simulink model "CryoDetXray"  (R2016b)
settings: Solver=ode45  StartTime=0.0  StopTime=10e-5  MaxStep=Tclk/4  RelTol=1e-3
values from neighbouring files (symbols this model uses):
  Fclk = Fadc    (= 307200000)    [setupCryoFPGAxray.m]
  Tclk = 1/Fclk    (= 3.25520833333e-09)    [setupCryoFPGAxray.m]
undefined symbols (not defined in the file or in its folder): AXI4, Lite, lpf, Naxi, xlipgetpartsetting
libraries: xbsIndex_r4 x1091, CryoDetLib x68, simulink x4, hdlsllib x1
(part 2 of 8)

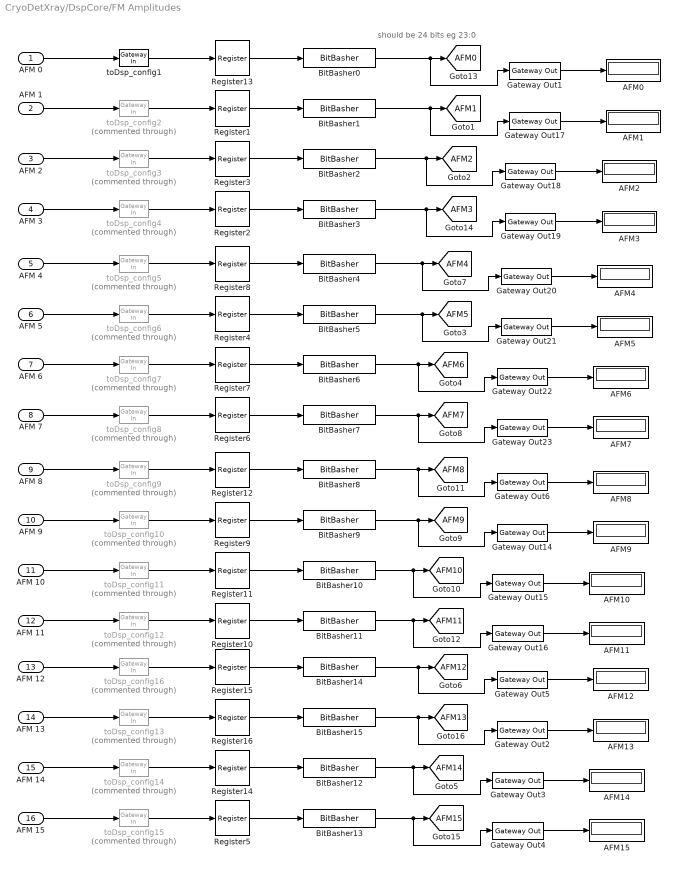
== system CryoDetXray/DspCore/FM Amplitudes ==
  note: should be 24 bits eg 23:0
  AFM 0 : Inport
  AFM 1 : Inport  Port=2
  AFM 2 : Inport  Port=3
  AFM 3 : Inport  Port=4
  AFM 4 : Inport  Port=5
  AFM 5 : Inport  Port=6
  AFM 6 : Inport  Port=7
  AFM 7 : Inport  Port=8
  AFM 8 : Inport  Port=9
  AFM 9 : Inport  Port=10
  AFM 10 : Inport  Port=11
  AFM 11 : Inport  Port=12
  AFM 12 : Inport  Port=13
  AFM 13 : Inport  Port=14
  AFM 14 : Inport  Port=15
  AFM 15 : Inport  Port=16
  AFM{0..5,7,9..15} (14 alike) : Display
  "AFM6 " : Display
  "AFM8 " : Display
  BitBasher{0..15} (16 alike) : xbsIndex_r4/BitBasher  bitexpr=a={b[23:0]}  display_expr=on  sr_1=a  arith_type1=Unsigned  bin_pt1=24  sr_2=2  arith_type2=Unsigned  bin_pt2=0  sr_3=3  arith_type3=Unsigned  bin_pt3=0  sr_4=4  arith_type4=Unsigned  bin_pt4=0  dbl_ovrd=off  block_type=bitbasher
  Gateway Out{1..6,14..23} (16 alike) : xbsIndex_r4/Gateway Out  inherit_from_input=on  hdl_port=off  rows=1  columns=1  UseAsDAC=off  DACChannel='1'  interface=None  automatic_assignment=on  address_offset=hex2dec('00')  intf_name=''  intf_description=''  timing_constraint=None  locs_specified=off  LOCs={}  io_standard={}  block_type=gatewayout
  Register{1..16} (16 alike) : xbsIndex_r4/Register  init=0  rst=off  en=off  dbl_ovrd=off  block_type=register
  toDsp_config1 : xbsIndex_r4/Gateway In  gui_display_data_type=Fixed-point  arith_type=Unsigned  n_bits=32  bin_pt=0  preci_type=Single  exp_width=8  frac_width=24  rows=1  columns=1  quantization=Truncate  overflow=Wrap  period=Tclk*Naxi  UseAsADC=off  ADCChannel='1'  interface=AXI4-Lite  automatic_assignment=off  address_offset=hex2dec('A00')  intf_name=''  intf_description=''  default_value=0  timing_constraint=None  locs_specified=off  LOCs={}  io_standard={}  inherit_from_input=off  hdl_port=on  dbl_ovrd=off  block_type=gatewayin
  toDsp_config10 : xbsIndex_r4/Gateway In  Commented=through  gui_display_data_type=Fixed-point  arith_type=Unsigned  n_bits=32  bin_pt=0  preci_type=Single  exp_width=8  frac_width=24  rows=1  columns=1  quantization=Truncate  overflow=Wrap  period=Tclk*Naxi  UseAsADC=off  ADCChannel='1'  interface=AXI4-Lite  automatic_assignment=off  address_offset=hex2dec('A24')  intf_name=''  intf_description=''  default_value=0  timing_constraint=None  locs_specified=off  LOCs={}  io_standard={}  inherit_from_input=off  hdl_port=on  dbl_ovrd=off  block_type=gatewayin
  toDsp_config11 : xbsIndex_r4/Gateway In  Commented=through  gui_display_data_type=Fixed-point  arith_type=Unsigned  n_bits=32  bin_pt=0  preci_type=Single  exp_width=8  frac_width=24  rows=1  columns=1  quantization=Truncate  overflow=Wrap  period=Tclk*Naxi  UseAsADC=off  ADCChannel='1'  interface=AXI4-Lite  automatic_assignment=off  address_offset=hex2dec('A28')  intf_name=''  intf_description=''  default_value=0  timing_constraint=None  locs_specified=off  LOCs={}  io_standard={}  inherit_from_input=off  hdl_port=on  dbl_ovrd=off  block_type=gatewayin
  toDsp_config12 : xbsIndex_r4/Gateway In  Commented=through  gui_display_data_type=Fixed-point  arith_type=Unsigned  n_bits=32  bin_pt=0  preci_type=Single  exp_width=8  frac_width=24  rows=1  columns=1  quantization=Truncate  overflow=Wrap  period=Tclk*Naxi  UseAsADC=off  ADCChannel='1'  interface=AXI4-Lite  automatic_assignment=off  address_offset=hex2dec('A2c')  intf_name=''  intf_description=''  default_value=0  timing_constraint=None  locs_specified=off  LOCs={}  io_standard={}  inherit_from_input=off  hdl_port=on  dbl_ovrd=off  block_type=gatewayin
  toDsp_config13 : xbsIndex_r4/Gateway In  Commented=through  gui_display_data_type=Fixed-point  arith_type=Unsigned  n_bits=32  bin_pt=0  preci_type=Single  exp_width=8  frac_width=24  rows=1  columns=1  quantization=Truncate  overflow=Wrap  period=Tclk*Naxi  UseAsADC=off  ADCChannel='1'  interface=AXI4-Lite  automatic_assignment=off  address_offset=hex2dec('A34')  intf_name=''  intf_description=''  default_value=0  timing_constraint=None  locs_specified=off  LOCs={}  io_standard={}  inherit_from_input=off  hdl_port=on  dbl_ovrd=off  block_type=gatewayin
  toDsp_config14 : xbsIndex_r4/Gateway In  Commented=through  gui_display_data_type=Fixed-point  arith_type=Unsigned  n_bits=32  bin_pt=0  preci_type=Single  exp_width=8  frac_width=24  rows=1  columns=1  quantization=Truncate  overflow=Wrap  period=Tclk*Naxi  UseAsADC=off  ADCChannel='1'  interface=AXI4-Lite  automatic_assignment=off  address_offset=hex2dec('A38')  intf_name=''  intf_description=''  default_value=0  timing_constraint=None  locs_specified=off  LOCs={}  io_standard={}  inherit_from_input=off  hdl_port=on  dbl_ovrd=off  block_type=gatewayin
  toDsp_config15 : xbsIndex_r4/Gateway In  Commented=through  gui_display_data_type=Fixed-point  arith_type=Unsigned  n_bits=32  bin_pt=0  preci_type=Single  exp_width=8  frac_width=24  rows=1  columns=1  quantization=Truncate  overflow=Wrap  period=Tclk*Naxi  UseAsADC=off  ADCChannel='1'  interface=AXI4-Lite  automatic_assignment=off  address_offset=hex2dec('A3c')  intf_name=''  intf_description=''  default_value=0  timing_constraint=None  locs_specified=off  LOCs={}  io_standard={}  inherit_from_input=off  hdl_port=on  dbl_ovrd=off  block_type=gatewayin
  toDsp_config16 : xbsIndex_r4/Gateway In  Commented=through  gui_display_data_type=Fixed-point  arith_type=Unsigned  n_bits=32  bin_pt=0  preci_type=Single  exp_width=8  frac_width=24  rows=1  columns=1  quantization=Truncate  overflow=Wrap  period=Tclk*Naxi  UseAsADC=off  ADCChannel='1'  interface=AXI4-Lite  automatic_assignment=off  address_offset=hex2dec('A30')  intf_name=''  intf_description=''  default_value=0  timing_constraint=None  locs_specified=off  LOCs={}  io_standard={}  inherit_from_input=off  hdl_port=on  dbl_ovrd=off  block_type=gatewayin
  toDsp_config2 : xbsIndex_r4/Gateway In  Commented=through  gui_display_data_type=Fixed-point  arith_type=Unsigned  n_bits=32  bin_pt=0  preci_type=Single  exp_width=8  frac_width=24  rows=1  columns=1  quantization=Truncate  overflow=Wrap  period=Tclk*Naxi  UseAsADC=off  ADCChannel='1'  interface=AXI4-Lite  automatic_assignment=off  address_offset=hex2dec('A04')  intf_name=''  intf_description=''  default_value=0  timing_constraint=None  locs_specified=off  LOCs={}  io_standard={}  inherit_from_input=off  hdl_port=on  dbl_ovrd=off  block_type=gatewayin
  toDsp_config3 : xbsIndex_r4/Gateway In  Commented=through  gui_display_data_type=Fixed-point  arith_type=Unsigned  n_bits=32  bin_pt=0  preci_type=Single  exp_width=8  frac_width=24  rows=1  columns=1  quantization=Truncate  overflow=Wrap  period=Tclk*Naxi  UseAsADC=off  ADCChannel='1'  interface=AXI4-Lite  automatic_assignment=off  address_offset=hex2dec('A08')  intf_name=''  intf_description=''  default_value=0  timing_constraint=None  locs_specified=off  LOCs={}  io_standard={}  inherit_from_input=off  hdl_port=on  dbl_ovrd=off  block_type=gatewayin
  toDsp_config4 : xbsIndex_r4/Gateway In  Commented=through  gui_display_data_type=Fixed-point  arith_type=Unsigned  n_bits=32  bin_pt=0  preci_type=Single  exp_width=8  frac_width=24  rows=1  columns=1  quantization=Truncate  overflow=Wrap  period=Tclk*Naxi  UseAsADC=off  ADCChannel='1'  interface=AXI4-Lite  automatic_assignment=off  address_offset=hex2dec('A0c')  intf_name=''  intf_description=''  default_value=0  timing_constraint=None  locs_specified=off  LOCs={}  io_standard={}  inherit_from_input=off  hdl_port=on  dbl_ovrd=off  block_type=gatewayin
  toDsp_config5 : xbsIndex_r4/Gateway In  Commented=through  gui_display_data_type=Fixed-point  arith_type=Unsigned  n_bits=32  bin_pt=0  preci_type=Single  exp_width=8  frac_width=24  rows=1  columns=1  quantization=Truncate  overflow=Wrap  period=Tclk*Naxi  UseAsADC=off  ADCChannel='1'  interface=AXI4-Lite  automatic_assignment=off  address_offset=hex2dec('A10')  intf_name=''  intf_description=''  default_value=0  timing_constraint=None  locs_specified=off  LOCs={}  io_standard={}  inherit_from_input=off  hdl_port=on  dbl_ovrd=off  block_type=gatewayin
  toDsp_config6 : xbsIndex_r4/Gateway In  Commented=through  gui_display_data_type=Fixed-point  arith_type=Unsigned  n_bits=32  bin_pt=0  preci_type=Single  exp_width=8  frac_width=24  rows=1  columns=1  quantization=Truncate  overflow=Wrap  period=Tclk*Naxi  UseAsADC=off  ADCChannel='1'  interface=AXI4-Lite  automatic_assignment=off  address_offset=hex2dec('A14')  intf_name=''  intf_description=''  default_value=0  timing_constraint=None  locs_specified=off  LOCs={}  io_standard={}  inherit_from_input=off  hdl_port=on  dbl_ovrd=off  block_type=gatewayin
  toDsp_config7 : xbsIndex_r4/Gateway In  Commented=through  gui_display_data_type=Fixed-point  arith_type=Unsigned  n_bits=32  bin_pt=0  preci_type=Single  exp_width=8  frac_width=24  rows=1  columns=1  quantization=Truncate  overflow=Wrap  period=Tclk*Naxi  UseAsADC=off  ADCChannel='1'  interface=AXI4-Lite  automatic_assignment=off  address_offset=hex2dec('A18')  intf_name=''  intf_description=''  default_value=0  timing_constraint=None  locs_specified=off  LOCs={}  io_standard={}  inherit_from_input=off  hdl_port=on  dbl_ovrd=off  block_type=gatewayin
  toDsp_config8 : xbsIndex_r4/Gateway In  Commented=through  gui_display_data_type=Fixed-point  arith_type=Unsigned  n_bits=32  bin_pt=0  preci_type=Single  exp_width=8  frac_width=24  rows=1  columns=1  quantization=Truncate  overflow=Wrap  period=Tclk*Naxi  UseAsADC=off  ADCChannel='1'  interface=AXI4-Lite  automatic_assignment=off  address_offset=hex2dec('A1c')  intf_name=''  intf_description=''  default_value=0  timing_constraint=None  locs_specified=off  LOCs={}  io_standard={}  inherit_from_input=off  hdl_port=on  dbl_ovrd=off  block_type=gatewayin
  toDsp_config9 : xbsIndex_r4/Gateway In  Commented=through  gui_display_data_type=Fixed-point  arith_type=Unsigned  n_bits=32  bin_pt=0  preci_type=Single  exp_width=8  frac_width=24  rows=1  columns=1  quantization=Truncate  overflow=Wrap  period=Tclk*Naxi  UseAsADC=off  ADCChannel='1'  interface=AXI4-Lite  automatic_assignment=off  address_offset=hex2dec('A20')  intf_name=''  intf_description=''  default_value=0  timing_constraint=None  locs_specified=off  LOCs={}  io_standard={}  inherit_from_input=off  hdl_port=on  dbl_ovrd=off  block_type=gatewayin
  tag scope: AFM0=global, AFM10=global, AFM11=global, AFM12=global, AFM13=global, AFM14=global, AFM15=global, AFM1=global, AFM2=global, AFM3=global, AFM4=global, AFM5=global, AFM6=global, AFM7=global, AFM8=global, AFM9=global
  wires:
  Gateway Out14/1 -> AFM9/1
  AFM 10/1 -> toDsp_config11/1
  toDsp_config11/1 -> Register11/1
  Register4/1 -> BitBasher5/1
  BitBasher11/1 -> Gateway Out16/1, [AFM11]
  Register10/1 -> BitBasher11/1
  toDsp_config6/1 -> Register4/1
  Gateway Out20/1 -> AFM4/1
  BitBasher4/1 -> Gateway Out20/1, [AFM4]
  toDsp_config1/1 -> Register13/1
  Gateway Out15/1 -> AFM10/1
  Register11/1 -> BitBasher10/1
  BitBasher10/1 -> Gateway Out15/1, [AFM10]
  AFM 0/1 -> toDsp_config1/1
  Gateway Out22/1 -> "AFM6 "/1
  AFM 7/1 -> toDsp_config8/1
  toDsp_config8/1 -> Register6/1
  Gateway Out1/1 -> AFM0/1
  Register2/1 -> BitBasher3/1
  Gateway Out18/1 -> AFM2/1
  BitBasher2/1 -> Gateway Out18/1, [AFM2]
  Gateway Out19/1 -> AFM3/1
  BitBasher3/1 -> Gateway Out19/1, [AFM3]
  Register6/1 -> BitBasher7/1
  Gateway Out6/1 -> "AFM8 "/1
  Register9/1 -> BitBasher9/1
  AFM 2/1 -> toDsp_config3/1
  toDsp_config3/1 -> Register3/1
  Gateway Out23/1 -> AFM7/1
  BitBasher1/1 -> Gateway Out17/1, [AFM1]
  BitBasher6/1 -> Gateway Out22/1, [AFM6]
  toDsp_config2/1 -> Register1/1
  AFM 1/1 -> toDsp_config2/1
  Register12/1 -> BitBasher8/1
  Gateway Out16/1 -> AFM11/1
  Gateway Out21/1 -> AFM5/1
  BitBasher5/1 -> Gateway Out21/1, [AFM5]
  BitBasher7/1 -> Gateway Out23/1, [AFM7]
  BitBasher0/1 -> Gateway Out1/1, [AFM0]
  AFM 5/1 -> toDsp_config6/1
  BitBasher8/1 -> Gateway Out6/1, [AFM8]
  Register7/1 -> BitBasher6/1
  BitBasher9/1 -> Gateway Out14/1, [AFM9]
  AFM 8/1 -> toDsp_config9/1
  toDsp_config9/1 -> Register12/1
  AFM 6/1 -> toDsp_config7/1
  toDsp_config7/1 -> Register7/1
  AFM 11/1 -> toDsp_config12/1
  toDsp_config12/1 -> Register10/1
  AFM 9/1 -> toDsp_config10/1
  toDsp_config10/1 -> Register9/1
  Register13/1 -> BitBasher0/1
  Register8/1 -> BitBasher4/1
  toDsp_config5/1 -> Register8/1
  AFM 4/1 -> toDsp_config5/1
  Register1/1 -> BitBasher1/1
  Gateway Out17/1 -> AFM1/1
  Register3/1 -> BitBasher2/1
  AFM 3/1 -> toDsp_config4/1
  toDsp_config4/1 -> Register2/1
  Gateway Out2/1 -> AFM13/1
  AFM 14/1 -> toDsp_config14/1
  toDsp_config14/1 -> Register14/1
  BitBasher13/1 -> Gateway Out4/1, [AFM15]
  Register5/1 -> BitBasher13/1
  Gateway Out3/1 -> AFM14/1
  Register14/1 -> BitBasher12/1
  BitBasher12/1 -> Gateway Out3/1, [AFM14]
  Gateway Out5/1 -> AFM12/1
  Register16/1 -> BitBasher15/1
  Register15/1 -> BitBasher14/1
  Gateway Out4/1 -> AFM15/1
  BitBasher14/1 -> Gateway Out5/1, [AFM12]
  BitBasher15/1 -> Gateway Out2/1, [AFM13]
  AFM 12/1 -> toDsp_config16/1
  toDsp_config16/1 -> Register15/1
  AFM 15/1 -> toDsp_config15/1
  toDsp_config15/1 -> Register5/1
  AFM 13/1 -> toDsp_config13/1
  toDsp_config13/1 -> Register16/1

== system CryoDetXray/DspCore/FRreset ==
  note: FluxRampReset
      | One shot to trigger reset of flux ramp generator
      | Constant5 sets number of clocks in high state
  FRreset : Inport
  Constant1 : xbsIndex_r4/Constant  const=0  gui_display_data_type=Fixed-point  arith_type=Unsigned  n_bits=8  bin_pt=0  preci_type=Single  exp_width=8  frac_width=24  explicit_period=off  period=1  equ=P=C  opselect=C  inp2=PCIN>>17  opr=+  inp1=P  carry=CIN  dbl_ovrd=off  block_type=constant
  Constant2 : xbsIndex_r4/Constant  const=45  gui_display_data_type=Fixed-point  arith_type=Unsigned  n_bits=8  bin_pt=0  preci_type=Single  exp_width=8  frac_width=24  explicit_period=off  period=1  equ=P=C  opselect=C  inp2=PCIN>>17  opr=+  inp1=P  carry=CIN  dbl_ovrd=off  block_type=constant
  Convert : xbsIndex_r4/Convert  gui_display_data_type=Fixed-point  arith_type=Unsigned  n_bits=16  bin_pt=0  float_type=Single  exp_bits=8  fraction_bits=24  quantization=Truncate  overflow=Wrap  en=off  latency=1  pipeline=off  dbl_ovrd=off  block_type=convert
  Counter1 : xbsIndex_r4/Counter  cnt_type=Count Limited  cnt_to=255  operation=Up  start_count=0  cnt_by_val=1  arith_type=Unsigned  n_bits=8  bin_pt=0  load_pin=on  rst=on  en=off  explicit_period=off  period=5e-9  use_behavioral_HDL=off  implementation=Fabric  dbl_ovrd=off  block_type=counter
  Expression : xbsIndex_r4/Expression  expression=ready & ~start | finish  align_bp=on  en=off  latency=0  precision=Full  arith_type=Unsigned  n_bits=16  bin_pt=0  dbl_ovrd=off  block_type=expr
  Flux Ramp Reset Scope : Scope  NumInputPorts=2
  Gateway Out : xbsIndex_r4/Gateway Out  inherit_from_input=off  hdl_port=off  rows=1  columns=1  UseAsDAC=off  DACChannel='1'  interface=None  automatic_assignment=on  address_offset=hex2dec('00')  intf_name=''  intf_description=''  timing_constraint=None  locs_specified=off  LOCs={}  io_standard={}  block_type=gatewayout
  Gateway Out1 : xbsIndex_r4/Gateway Out  inherit_from_input=off  hdl_port=off  rows=1  columns=1  UseAsDAC=off  DACChannel='1'  interface=None  automatic_assignment=on  address_offset=hex2dec('00')  intf_name=''  intf_description=''  timing_constraint=None  locs_specified=off  LOCs={}  io_standard={}  block_type=gatewayout
  Inverter : xbsIndex_r4/Inverter  en=off  latency=0  dbl_ovrd=off  block_type=inv
  Register : xbsIndex_r4/Register  init=0  rst=off  en=off  dbl_ovrd=off  block_type=register
  Relational1 : xbsIndex_r4/Relational  mode=a=b  op_type=Bool  en=off  latency=0  dbl_ovrd=off  block_type=relational
  Relational2 : xbsIndex_r4/Relational  mode=a>b  op_type=Bool  en=off  latency=0  dbl_ovrd=off  block_type=relational
  Out1 : Outport
  wires:
  Counter1/1 -> Relational2/1, Relational1/2
  Constant1/1 -> Relational1/1
  Constant2/1 -> Relational2/2
  FRreset/1 -> Gateway Out/1, Expression/3
  Relational2/1 -> Expression/1
  Relational1/1 -> Inverter/1, Expression/2
  Expression/1 -> Counter1/1
  Inverter/1 -> Gateway Out1/1, Convert/1
  Gateway Out/1 -> Flux Ramp Reset Scope/1
  Gateway Out1/1 -> Flux Ramp Reset Scope/2
  Convert/1 -> Register/1
  Register/1 -> Out1/1

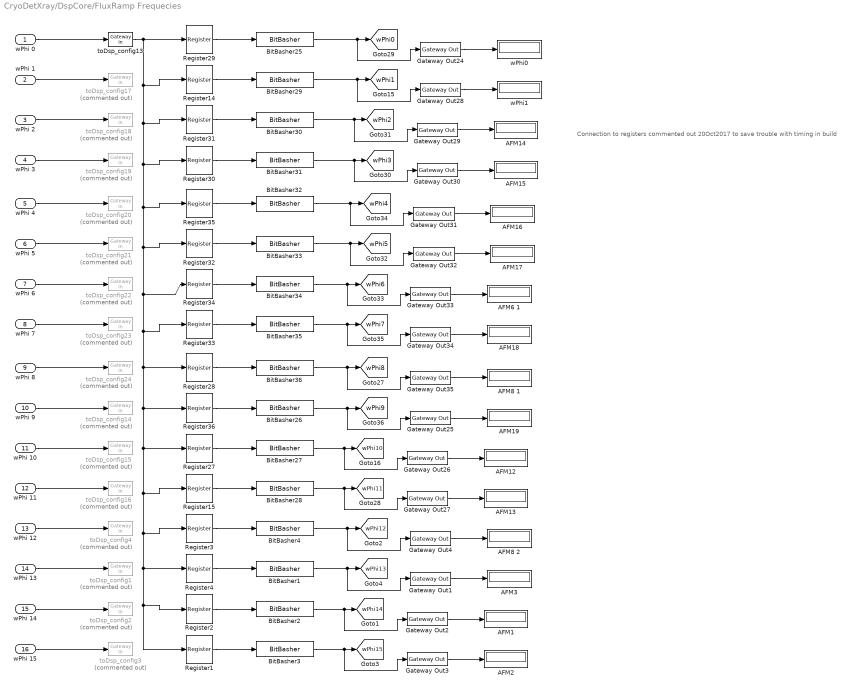
== system CryoDetXray/DspCore/FluxRamp Frequecies ==
  note: Connection to registers commented out 20Oct2017 to save trouble with timing in build
  wPhi 0 : Inport
  wPhi 1 : Inport  Port=2
  wPhi 2 : Inport  Port=3
  wPhi 3 : Inport  Port=4
  wPhi 4 : Inport  Port=5
  wPhi 5 : Inport  Port=6
  wPhi 6 : Inport  Port=7
  wPhi 7 : Inport  Port=8
  wPhi 8 : Inport  Port=9
  wPhi 9 : Inport  Port=10
  wPhi 10 : Inport  Port=11
  wPhi 11 : Inport  Port=12
  wPhi 12 : Inport  Port=13
  wPhi 13 : Inport  Port=14
  wPhi 14 : Inport  Port=15
  wPhi 15 : Inport  Port=16
  AFM{1..3,12..19} (11 alike) : Display
  AFM6 1 : Display
  AFM8 1 : Display
  AFM8 2 : Display
  BitBasher{1..4,25..36} (16 alike) : xbsIndex_r4/BitBasher  bitexpr=a={b[15:0]}  display_expr=on  sr_1=a  arith_type1=Unsigned  bin_pt1=16  sr_2=2  arith_type2=Unsigned  bin_pt2=0  sr_3=3  arith_type3=Unsigned  bin_pt3=0  sr_4=4  arith_type4=Unsigned  bin_pt4=0  dbl_ovrd=off  block_type=bitbasher
  Gateway Out{1..4,24..35} (16 alike) : xbsIndex_r4/Gateway Out  inherit_from_input=on  hdl_port=off  rows=1  columns=1  UseAsDAC=off  DACChannel='1'  interface=None  automatic_assignment=on  address_offset=hex2dec('00')  intf_name=''  intf_description=''  timing_constraint=None  locs_specified=off  LOCs={}  io_standard={}  block_type=gatewayout
  Register{1..4,14..15,27..36} (16 alike) : xbsIndex_r4/Register  init=0  rst=off  en=off  dbl_ovrd=off  block_type=register
  toDsp_config1 : xbsIndex_r4/Gateway In  Commented=on  gui_display_data_type=Fixed-point  arith_type=Unsigned  n_bits=32  bin_pt=0  preci_type=Single  exp_width=8  frac_width=24  rows=1  columns=1  quantization=Truncate  overflow=Wrap  period=Tclk*Naxi  UseAsADC=off  ADCChannel='1'  interface=AXI4-Lite  automatic_assignment=off  address_offset=hex2dec('B34')  intf_name=''  intf_description=''  default_value=0  timing_constraint=None  locs_specified=off  LOCs={}  io_standard={}  inherit_from_input=off  hdl_port=on  dbl_ovrd=off  block_type=gatewayin
  toDsp_config13 : xbsIndex_r4/Gateway In  gui_display_data_type=Fixed-point  arith_type=Unsigned  n_bits=32  bin_pt=0  preci_type=Single  exp_width=8  frac_width=24  rows=1  columns=1  quantization=Truncate  overflow=Wrap  period=Tclk*Naxi  UseAsADC=off  ADCChannel='1'  interface=AXI4-Lite  automatic_assignment=off  address_offset=hex2dec('B00')  intf_name=''  intf_description=''  default_value=0  timing_constraint=None  locs_specified=off  LOCs={}  io_standard={}  inherit_from_input=off  hdl_port=on  dbl_ovrd=off  block_type=gatewayin
  toDsp_config14 : xbsIndex_r4/Gateway In  Commented=on  gui_display_data_type=Fixed-point  arith_type=Unsigned  n_bits=32  bin_pt=0  preci_type=Single  exp_width=8  frac_width=24  rows=1  columns=1  quantization=Truncate  overflow=Wrap  period=Tclk*Naxi  UseAsADC=off  ADCChannel='1'  interface=AXI4-Lite  automatic_assignment=off  address_offset=hex2dec('B24')  intf_name=''  intf_description=''  default_value=0  timing_constraint=None  locs_specified=off  LOCs={}  io_standard={}  inherit_from_input=off  hdl_port=on  dbl_ovrd=off  block_type=gatewayin
  toDsp_config15 : xbsIndex_r4/Gateway In  Commented=on  gui_display_data_type=Fixed-point  arith_type=Unsigned  n_bits=32  bin_pt=0  preci_type=Single  exp_width=8  frac_width=24  rows=1  columns=1  quantization=Truncate  overflow=Wrap  period=Tclk*Naxi  UseAsADC=off  ADCChannel='1'  interface=AXI4-Lite  automatic_assignment=off  address_offset=hex2dec('B28')  intf_name=''  intf_description=''  default_value=0  timing_constraint=None  locs_specified=off  LOCs={}  io_standard={}  inherit_from_input=off  hdl_port=on  dbl_ovrd=off  block_type=gatewayin
  toDsp_config16 : xbsIndex_r4/Gateway In  Commented=on  gui_display_data_type=Fixed-point  arith_type=Unsigned  n_bits=32  bin_pt=0  preci_type=Single  exp_width=8  frac_width=24  rows=1  columns=1  quantization=Truncate  overflow=Wrap  period=Tclk*Naxi  UseAsADC=off  ADCChannel='1'  interface=AXI4-Lite  automatic_assignment=off  address_offset=hex2dec('B2c')  intf_name=''  intf_description=''  default_value=0  timing_constraint=None  locs_specified=off  LOCs={}  io_standard={}  inherit_from_input=off  hdl_port=on  dbl_ovrd=off  block_type=gatewayin
  toDsp_config17 : xbsIndex_r4/Gateway In  Commented=on  gui_display_data_type=Fixed-point  arith_type=Unsigned  n_bits=32  bin_pt=0  preci_type=Single  exp_width=8  frac_width=24  rows=1  columns=1  quantization=Truncate  overflow=Wrap  period=Tclk*Naxi  UseAsADC=off  ADCChannel='1'  interface=AXI4-Lite  automatic_assignment=off  address_offset=hex2dec('B04')  intf_name=''  intf_description=''  default_value=0  timing_constraint=None  locs_specified=off  LOCs={}  io_standard={}  inherit_from_input=off  hdl_port=on  dbl_ovrd=off  block_type=gatewayin
  toDsp_config18 : xbsIndex_r4/Gateway In  Commented=on  gui_display_data_type=Fixed-point  arith_type=Unsigned  n_bits=32  bin_pt=0  preci_type=Single  exp_width=8  frac_width=24  rows=1  columns=1  quantization=Truncate  overflow=Wrap  period=Tclk*Naxi  UseAsADC=off  ADCChannel='1'  interface=AXI4-Lite  automatic_assignment=off  address_offset=hex2dec('b08')  intf_name=''  intf_description=''  default_value=0  timing_constraint=None  locs_specified=off  LOCs={}  io_standard={}  inherit_from_input=off  hdl_port=on  dbl_ovrd=off  block_type=gatewayin
  toDsp_config19 : xbsIndex_r4/Gateway In  Commented=on  gui_display_data_type=Fixed-point  arith_type=Unsigned  n_bits=32  bin_pt=0  preci_type=Single  exp_width=8  frac_width=24  rows=1  columns=1  quantization=Truncate  overflow=Wrap  period=Tclk*Naxi  UseAsADC=off  ADCChannel='1'  interface=AXI4-Lite  automatic_assignment=off  address_offset=hex2dec('b0c')  intf_name=''  intf_description=''  default_value=0  timing_constraint=None  locs_specified=off  LOCs={}  io_standard={}  inherit_from_input=off  hdl_port=on  dbl_ovrd=off  block_type=gatewayin
  toDsp_config2 : xbsIndex_r4/Gateway In  Commented=on  gui_display_data_type=Fixed-point  arith_type=Unsigned  n_bits=32  bin_pt=0  preci_type=Single  exp_width=8  frac_width=24  rows=1  columns=1  quantization=Truncate  overflow=Wrap  period=Tclk*Naxi  UseAsADC=off  ADCChannel='1'  interface=AXI4-Lite  automatic_assignment=off  address_offset=hex2dec('B38')  intf_name=''  intf_description=''  default_value=0  timing_constraint=None  locs_specified=off  LOCs={}  io_standard={}  inherit_from_input=off  hdl_port=on  dbl_ovrd=off  block_type=gatewayin
  toDsp_config20 : xbsIndex_r4/Gateway In  Commented=on  gui_display_data_type=Fixed-point  arith_type=Unsigned  n_bits=32  bin_pt=0  preci_type=Single  exp_width=8  frac_width=24  rows=1  columns=1  quantization=Truncate  overflow=Wrap  period=Tclk*Naxi  UseAsADC=off  ADCChannel='1'  interface=AXI4-Lite  automatic_assignment=off  address_offset=hex2dec('B10')  intf_name=''  intf_description=''  default_value=0  timing_constraint=None  locs_specified=off  LOCs={}  io_standard={}  inherit_from_input=off  hdl_port=on  dbl_ovrd=off  block_type=gatewayin
  toDsp_config21 : xbsIndex_r4/Gateway In  Commented=on  gui_display_data_type=Fixed-point  arith_type=Unsigned  n_bits=32  bin_pt=0  preci_type=Single  exp_width=8  frac_width=24  rows=1  columns=1  quantization=Truncate  overflow=Wrap  period=Tclk*Naxi  UseAsADC=off  ADCChannel='1'  interface=AXI4-Lite  automatic_assignment=off  address_offset=hex2dec('B14')  intf_name=''  intf_description=''  default_value=0  timing_constraint=None  locs_specified=off  LOCs={}  io_standard={}  inherit_from_input=off  hdl_port=on  dbl_ovrd=off  block_type=gatewayin
  toDsp_config22 : xbsIndex_r4/Gateway In  Commented=on  gui_display_data_type=Fixed-point  arith_type=Unsigned  n_bits=32  bin_pt=0  preci_type=Single  exp_width=8  frac_width=24  rows=1  columns=1  quantization=Truncate  overflow=Wrap  period=Tclk*Naxi  UseAsADC=off  ADCChannel='1'  interface=AXI4-Lite  automatic_assignment=off  address_offset=hex2dec('B18')  intf_name=''  intf_description=''  default_value=0  timing_constraint=None  locs_specified=off  LOCs={}  io_standard={}  inherit_from_input=off  hdl_port=on  dbl_ovrd=off  block_type=gatewayin
  toDsp_config23 : xbsIndex_r4/Gateway In  Commented=on  gui_display_data_type=Fixed-point  arith_type=Unsigned  n_bits=32  bin_pt=0  preci_type=Single  exp_width=8  frac_width=24  rows=1  columns=1  quantization=Truncate  overflow=Wrap  period=Tclk*Naxi  UseAsADC=off  ADCChannel='1'  interface=AXI4-Lite  automatic_assignment=off  address_offset=hex2dec('B1c')  intf_name=''  intf_description=''  default_value=0  timing_constraint=None  locs_specified=off  LOCs={}  io_standard={}  inherit_from_input=off  hdl_port=on  dbl_ovrd=off  block_type=gatewayin
  toDsp_config24 : xbsIndex_r4/Gateway In  Commented=on  gui_display_data_type=Fixed-point  arith_type=Unsigned  n_bits=32  bin_pt=0  preci_type=Single  exp_width=8  frac_width=24  rows=1  columns=1  quantization=Truncate  overflow=Wrap  period=Tclk*Naxi  UseAsADC=off  ADCChannel='1'  interface=AXI4-Lite  automatic_assignment=off  address_offset=hex2dec('B20')  intf_name=''  intf_description=''  default_value=0  timing_constraint=None  locs_specified=off  LOCs={}  io_standard={}  inherit_from_input=off  hdl_port=on  dbl_ovrd=off  block_type=gatewayin
  toDsp_config3 : xbsIndex_r4/Gateway In  Commented=on  gui_display_data_type=Fixed-point  arith_type=Unsigned  n_bits=32  bin_pt=0  preci_type=Single  exp_width=8  frac_width=24  rows=1  columns=1  quantization=Truncate  overflow=Wrap  period=Tclk*Naxi  UseAsADC=off  ADCChannel='1'  interface=AXI4-Lite  automatic_assignment=off  address_offset=hex2dec('B3c')  intf_name=''  intf_description=''  default_value=0  timing_constraint=None  locs_specified=off  LOCs={}  io_standard={}  inherit_from_input=off  hdl_port=on  dbl_ovrd=off  block_type=gatewayin
  toDsp_config4 : xbsIndex_r4/Gateway In  Commented=on  gui_display_data_type=Fixed-point  arith_type=Unsigned  n_bits=32  bin_pt=0  preci_type=Single  exp_width=8  frac_width=24  rows=1  columns=1  quantization=Truncate  overflow=Wrap  period=Tclk*Naxi  UseAsADC=off  ADCChannel='1'  interface=AXI4-Lite  automatic_assignment=off  address_offset=hex2dec('B30')  intf_name=''  intf_description=''  default_value=0  timing_constraint=None  locs_specified=off  LOCs={}  io_standard={}  inherit_from_input=off  hdl_port=on  dbl_ovrd=off  block_type=gatewayin
  wPhi0 : Display
  wPhi1 : Display
  tag scope: wPhi0=global, wPhi10=global, wPhi11=global, wPhi12=global, wPhi13=global, wPhi14=global, wPhi15=global, wPhi1=global, wPhi2=global, wPhi3=global, wPhi4=global, wPhi5=global, wPhi6=global, wPhi7=global, wPhi8=global, wPhi9=global
  wires:
  Gateway Out25/1 -> AFM19/1
  wPhi 10/1 -> toDsp_config15/1
  Register32/1 -> BitBasher33/1
  BitBasher28/1 -> Gateway Out27/1, [wPhi11]
  Register15/1 -> BitBasher28/1
  Gateway Out31/1 -> AFM16/1
  BitBasher32/1 -> Gateway Out31/1, [wPhi4]
  Gateway Out26/1 -> AFM12/1
  Register27/1 -> BitBasher27/1
  BitBasher27/1 -> Gateway Out26/1, [wPhi10]
  wPhi 0/1 -> toDsp_config13/1
  Gateway Out33/1 -> AFM6 1/1
  wPhi 7/1 -> toDsp_config23/1
  Gateway Out24/1 -> wPhi0/1
  Register30/1 -> BitBasher31/1
  Gateway Out29/1 -> AFM14/1
  BitBasher30/1 -> Gateway Out29/1, [wPhi2]
  Gateway Out30/1 -> AFM15/1
  BitBasher31/1 -> Gateway Out30/1, [wPhi3]
  Register33/1 -> BitBasher35/1
  Gateway Out35/1 -> AFM8 1/1
  Register36/1 -> BitBasher26/1
  wPhi 2/1 -> toDsp_config18/1
  Gateway Out34/1 -> AFM18/1
  BitBasher29/1 -> Gateway Out28/1, [wPhi1]
  BitBasher34/1 -> Gateway Out33/1, [wPhi6]
  wPhi 1/1 -> toDsp_config17/1
  Register28/1 -> BitBasher36/1
  Gateway Out27/1 -> AFM13/1
  Gateway Out32/1 -> AFM17/1
  BitBasher33/1 -> Gateway Out32/1, [wPhi5]
  BitBasher35/1 -> Gateway Out34/1, [wPhi7]
  BitBasher25/1 -> Gateway Out24/1, [wPhi0]
  wPhi 5/1 -> toDsp_config21/1
  BitBasher36/1 -> Gateway Out35/1, [wPhi8]
  Register34/1 -> BitBasher34/1
  BitBasher26/1 -> Gateway Out25/1, [wPhi9]
  wPhi 8/1 -> toDsp_config24/1
  wPhi 6/1 -> toDsp_config22/1
  wPhi 11/1 -> toDsp_config16/1
  wPhi 9/1 -> toDsp_config14/1
  Register29/1 -> BitBasher25/1
  Register35/1 -> BitBasher32/1
  wPhi 4/1 -> toDsp_config20/1
  Register14/1 -> BitBasher29/1
  Gateway Out28/1 -> wPhi1/1
  Register31/1 -> BitBasher30/1
  wPhi 3/1 -> toDsp_config19/1
  Gateway Out1/1 -> AFM3/1
  wPhi 14/1 -> toDsp_config2/1
  BitBasher3/1 -> Gateway Out3/1, [wPhi15]
  Register1/1 -> BitBasher3/1
  Gateway Out2/1 -> AFM1/1
  Register2/1 -> BitBasher2/1
  BitBasher2/1 -> Gateway Out2/1, [wPhi14]
  Gateway Out4/1 -> AFM8 2/1
  Register4/1 -> BitBasher1/1
  Register3/1 -> BitBasher4/1
  Gateway Out3/1 -> AFM2/1
  BitBasher4/1 -> Gateway Out4/1, [wPhi12]
  BitBasher1/1 -> Gateway Out1/1, [wPhi13]
  wPhi 12/1 -> toDsp_config4/1
  wPhi 15/1 -> toDsp_config3/1
  wPhi 13/1 -> toDsp_config1/1
  toDsp_config13/1 -> Register14/1, Register31/1, Register30/1, Register35/1, Register32/1, Register34/1, Register33/1, Register28/1, Register36/1, Register27/1, Register15/1, Register3/1, Register4/1, Register2/1, Register1/1, Register29/1

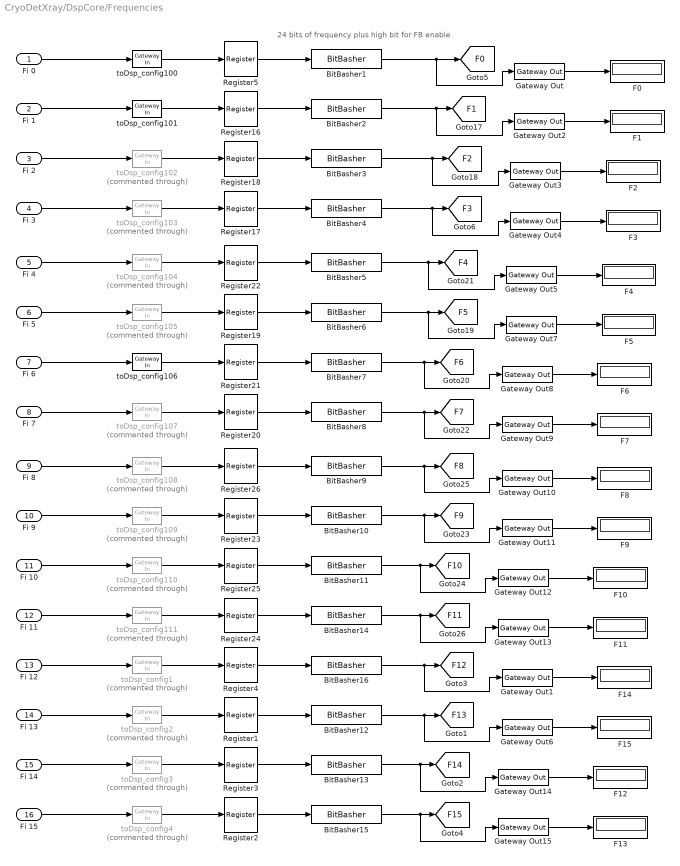
== system CryoDetXray/DspCore/Frequencies ==
  note: 24 bits of frequency plus high bit for FB enable
  "Fi 0 " : Inport
  Fi 1 : Inport  Port=2
  Fi 2 : Inport  Port=3
  Fi 3 : Inport  Port=4
  Fi 4 : Inport  Port=5
  Fi 5 : Inport  Port=6
  Fi 6 : Inport  Port=7
  Fi 7 : Inport  Port=8
  Fi 8 : Inport  Port=9
  Fi 9 : Inport  Port=10
  Fi 10 : Inport  Port=11
  Fi 11 : Inport  Port=12
  Fi 12 : Inport  Port=13
  Fi 13 : Inport  Port=14
  Fi 14 : Inport  Port=15
  Fi 15 : Inport  Port=16
  BitBasher{1..16} (16 alike) : xbsIndex_r4/BitBasher  bitexpr=a={b[24:0]}  display_expr=on  sr_1=a  arith_type1=Unsigned  bin_pt1=0  sr_2=2  arith_type2=Unsigned  bin_pt2=0  sr_3=3  arith_type3=Unsigned  bin_pt3=0  sr_4=4  arith_type4=Unsigned  bin_pt4=0  dbl_ovrd=off  block_type=bitbasher
  F{0..15} (16 alike) : Display
  Gateway Out{,1..15} (16 alike) : xbsIndex_r4/Gateway Out  inherit_from_input=on  hdl_port=off  rows=1  columns=1  UseAsDAC=off  DACChannel='1'  interface=None  automatic_assignment=on  address_offset=hex2dec('00')  intf_name=''  intf_description=''  timing_constraint=None  locs_specified=off  LOCs={}  io_standard={}  block_type=gatewayout
  Register{1..5,16..26} (16 alike) : xbsIndex_r4/Register  init=0  rst=off  en=off  dbl_ovrd=off  block_type=register
  toDsp_config1 : xbsIndex_r4/Gateway In  Commented=through  gui_display_data_type=Fixed-point  arith_type=Unsigned  n_bits=32  bin_pt=0  preci_type=Single  exp_width=8  frac_width=24  rows=1  columns=1  quantization=Truncate  overflow=Wrap  period=Tclk*Naxi  UseAsADC=off  ADCChannel='1'  interface=AXI4-Lite  automatic_assignment=off  address_offset=hex2dec('930')  intf_name=''  intf_description=''  default_value=0  timing_constraint=None  locs_specified=off  LOCs={}  io_standard={}  inherit_from_input=off  hdl_port=on  dbl_ovrd=off  block_type=gatewayin
  toDsp_config100 : xbsIndex_r4/Gateway In  gui_display_data_type=Fixed-point  arith_type=Unsigned  n_bits=32  bin_pt=0  preci_type=Single  exp_width=8  frac_width=24  rows=1  columns=1  quantization=Truncate  overflow=Wrap  period=Tclk*Naxi  UseAsADC=off  ADCChannel='1'  interface=AXI4-Lite  automatic_assignment=off  address_offset=hex2dec('900')  intf_name=''  intf_description=''  default_value=0  timing_constraint=None  locs_specified=off  LOCs={}  io_standard={}  inherit_from_input=off  hdl_port=on  dbl_ovrd=off  block_type=gatewayin
  toDsp_config101 : xbsIndex_r4/Gateway In  gui_display_data_type=Fixed-point  arith_type=Unsigned  n_bits=32  bin_pt=0  preci_type=Single  exp_width=8  frac_width=24  rows=1  columns=1  quantization=Truncate  overflow=Wrap  period=Tclk*Naxi  UseAsADC=off  ADCChannel='1'  interface=AXI4-Lite  automatic_assignment=off  address_offset=hex2dec('904')  intf_name=''  intf_description=''  default_value=0  timing_constraint=None  locs_specified=off  LOCs={}  io_standard={}  inherit_from_input=off  hdl_port=on  dbl_ovrd=off  block_type=gatewayin
  toDsp_config102 : xbsIndex_r4/Gateway In  Commented=through  gui_display_data_type=Fixed-point  arith_type=Unsigned  n_bits=32  bin_pt=0  preci_type=Single  exp_width=8  frac_width=24  rows=1  columns=1  quantization=Truncate  overflow=Wrap  period=Tclk*Naxi  UseAsADC=off  ADCChannel='1'  interface=AXI4-Lite  automatic_assignment=off  address_offset=hex2dec('908')  intf_name=''  intf_description=''  default_value=0  timing_constraint=None  locs_specified=off  LOCs={}  io_standard={}  inherit_from_input=off  hdl_port=on  dbl_ovrd=off  block_type=gatewayin
  toDsp_config103 : xbsIndex_r4/Gateway In  Commented=through  gui_display_data_type=Fixed-point  arith_type=Unsigned  n_bits=32  bin_pt=0  preci_type=Single  exp_width=8  frac_width=24  rows=1  columns=1  quantization=Truncate  overflow=Wrap  period=Tclk*Naxi  UseAsADC=off  ADCChannel='1'  interface=AXI4-Lite  automatic_assignment=off  address_offset=hex2dec('90c')  intf_name=''  intf_description=''  default_value=0  timing_constraint=None  locs_specified=off  LOCs={}  io_standard={}  inherit_from_input=off  hdl_port=on  dbl_ovrd=off  block_type=gatewayin
  toDsp_config104 : xbsIndex_r4/Gateway In  Commented=through  gui_display_data_type=Fixed-point  arith_type=Unsigned  n_bits=32  bin_pt=0  preci_type=Single  exp_width=8  frac_width=24  rows=1  columns=1  quantization=Truncate  overflow=Wrap  period=Tclk*Naxi  UseAsADC=off  ADCChannel='1'  interface=AXI4-Lite  automatic_assignment=off  address_offset=hex2dec('910')  intf_name=''  intf_description=''  default_value=0  timing_constraint=None  locs_specified=off  LOCs={}  io_standard={}  inherit_from_input=off  hdl_port=on  dbl_ovrd=off  block_type=gatewayin
  toDsp_config105 : xbsIndex_r4/Gateway In  Commented=through  gui_display_data_type=Fixed-point  arith_type=Unsigned  n_bits=32  bin_pt=0  preci_type=Single  exp_width=8  frac_width=24  rows=1  columns=1  quantization=Truncate  overflow=Wrap  period=Tclk*Naxi  UseAsADC=off  ADCChannel='1'  interface=AXI4-Lite  automatic_assignment=off  address_offset=hex2dec('914')  intf_name=''  intf_description=''  default_value=0  timing_constraint=None  locs_specified=off  LOCs={}  io_standard={}  inherit_from_input=off  hdl_port=on  dbl_ovrd=off  block_type=gatewayin
  toDsp_config106 : xbsIndex_r4/Gateway In  gui_display_data_type=Fixed-point  arith_type=Unsigned  n_bits=32  bin_pt=0  preci_type=Single  exp_width=8  frac_width=24  rows=1  columns=1  quantization=Truncate  overflow=Wrap  period=Tclk*Naxi  UseAsADC=off  ADCChannel='1'  interface=AXI4-Lite  automatic_assignment=off  address_offset=hex2dec('918')  intf_name=''  intf_description=''  default_value=0  timing_constraint=None  locs_specified=off  LOCs={}  io_standard={}  inherit_from_input=off  hdl_port=on  dbl_ovrd=off  block_type=gatewayin
  toDsp_config107 : xbsIndex_r4/Gateway In  Commented=through  gui_display_data_type=Fixed-point  arith_type=Unsigned  n_bits=32  bin_pt=0  preci_type=Single  exp_width=8  frac_width=24  rows=1  columns=1  quantization=Truncate  overflow=Wrap  period=Tclk*Naxi  UseAsADC=off  ADCChannel='1'  interface=AXI4-Lite  automatic_assignment=off  address_offset=hex2dec('91c')  intf_name=''  intf_description=''  default_value=0  timing_constraint=None  locs_specified=off  LOCs={}  io_standard={}  inherit_from_input=off  hdl_port=on  dbl_ovrd=off  block_type=gatewayin
  toDsp_config108 : xbsIndex_r4/Gateway In  Commented=through  gui_display_data_type=Fixed-point  arith_type=Unsigned  n_bits=32  bin_pt=0  preci_type=Single  exp_width=8  frac_width=24  rows=1  columns=1  quantization=Truncate  overflow=Wrap  period=Tclk*Naxi  UseAsADC=off  ADCChannel='1'  interface=AXI4-Lite  automatic_assignment=off  address_offset=hex2dec('920')  intf_name=''  intf_description=''  default_value=0  timing_constraint=None  locs_specified=off  LOCs={}  io_standard={}  inherit_from_input=off  hdl_port=on  dbl_ovrd=off  block_type=gatewayin
  toDsp_config109 : xbsIndex_r4/Gateway In  Commented=through  gui_display_data_type=Fixed-point  arith_type=Unsigned  n_bits=32  bin_pt=0  preci_type=Single  exp_width=8  frac_width=24  rows=1  columns=1  quantization=Truncate  overflow=Wrap  period=Tclk*Naxi  UseAsADC=off  ADCChannel='1'  interface=AXI4-Lite  automatic_assignment=off  address_offset=hex2dec('924')  intf_name=''  intf_description=''  default_value=0  timing_constraint=None  locs_specified=off  LOCs={}  io_standard={}  inherit_from_input=off  hdl_port=on  dbl_ovrd=off  block_type=gatewayin
  toDsp_config110 : xbsIndex_r4/Gateway In  Commented=through  gui_display_data_type=Fixed-point  arith_type=Unsigned  n_bits=32  bin_pt=0  preci_type=Single  exp_width=8  frac_width=24  rows=1  columns=1  quantization=Truncate  overflow=Wrap  period=Tclk*Naxi  UseAsADC=off  ADCChannel='1'  interface=AXI4-Lite  automatic_assignment=off  address_offset=hex2dec('928')  intf_name=''  intf_description=''  default_value=0  timing_constraint=None  locs_specified=off  LOCs={}  io_standard={}  inherit_from_input=off  hdl_port=on  dbl_ovrd=off  block_type=gatewayin
  toDsp_config111 : xbsIndex_r4/Gateway In  Commented=through  gui_display_data_type=Fixed-point  arith_type=Unsigned  n_bits=32  bin_pt=0  preci_type=Single  exp_width=8  frac_width=24  rows=1  columns=1  quantization=Truncate  overflow=Wrap  period=Tclk*Naxi  UseAsADC=off  ADCChannel='1'  interface=AXI4-Lite  automatic_assignment=off  address_offset=hex2dec('92c')  intf_name=''  intf_description=''  default_value=0  timing_constraint=None  locs_specified=off  LOCs={}  io_standard={}  inherit_from_input=off  hdl_port=on  dbl_ovrd=off  block_type=gatewayin
  toDsp_config2 : xbsIndex_r4/Gateway In  Commented=through  gui_display_data_type=Fixed-point  arith_type=Unsigned  n_bits=32  bin_pt=0  preci_type=Single  exp_width=8  frac_width=24  rows=1  columns=1  quantization=Truncate  overflow=Wrap  period=Tclk*Naxi  UseAsADC=off  ADCChannel='1'  interface=AXI4-Lite  automatic_assignment=off  address_offset=hex2dec('934')  intf_name=''  intf_description=''  default_value=0  timing_constraint=None  locs_specified=off  LOCs={}  io_standard={}  inherit_from_input=off  hdl_port=on  dbl_ovrd=off  block_type=gatewayin
  toDsp_config3 : xbsIndex_r4/Gateway In  Commented=through  gui_display_data_type=Fixed-point  arith_type=Unsigned  n_bits=32  bin_pt=0  preci_type=Single  exp_width=8  frac_width=24  rows=1  columns=1  quantization=Truncate  overflow=Wrap  period=Tclk*Naxi  UseAsADC=off  ADCChannel='1'  interface=AXI4-Lite  automatic_assignment=off  address_offset=hex2dec('938')  intf_name=''  intf_description=''  default_value=0  timing_constraint=None  locs_specified=off  LOCs={}  io_standard={}  inherit_from_input=off  hdl_port=on  dbl_ovrd=off  block_type=gatewayin
  toDsp_config4 : xbsIndex_r4/Gateway In  Commented=through  gui_display_data_type=Fixed-point  arith_type=Unsigned  n_bits=32  bin_pt=0  preci_type=Single  exp_width=8  frac_width=24  rows=1  columns=1  quantization=Truncate  overflow=Wrap  period=Tclk*Naxi  UseAsADC=off  ADCChannel='1'  interface=AXI4-Lite  automatic_assignment=off  address_offset=hex2dec('93c')  intf_name=''  intf_description=''  default_value=0  timing_constraint=None  locs_specified=off  LOCs={}  io_standard={}  inherit_from_input=off  hdl_port=on  dbl_ovrd=off  block_type=gatewayin
  tag scope: F0=global, F10=global, F11=global, F12=global, F13=global, F14=global, F15=global, F1=global, F2=global, F3=global, F4=global, F5=global, F6=global, F7=global, F8=global, F9=global
  wires:
  Gateway Out11/1 -> F9/1
  Fi 10/1 -> toDsp_config110/1
  toDsp_config110/1 -> Register25/1
  Register19/1 -> BitBasher6/1
  BitBasher14/1 -> Gateway Out13/1, [F11]
  Register24/1 -> BitBasher14/1
  toDsp_config105/1 -> Register19/1
  Gateway Out5/1 -> F4/1
  BitBasher5/1 -> Gateway Out5/1, [F4]
  toDsp_config100/1 -> Register5/1
  Gateway Out12/1 -> F10/1
  Register25/1 -> BitBasher11/1
  BitBasher11/1 -> Gateway Out12/1, [F10]
  "Fi 0 "/1 -> toDsp_config100/1
  Gateway Out8/1 -> F6/1
  Fi 7/1 -> toDsp_config107/1
  toDsp_config107/1 -> Register20/1
  Gateway Out/1 -> F0/1
  Register17/1 -> BitBasher4/1
  Gateway Out3/1 -> F2/1
  BitBasher3/1 -> Gateway Out3/1, [F2]
  Gateway Out4/1 -> F3/1
  BitBasher4/1 -> Gateway Out4/1, [F3]
  Register20/1 -> BitBasher8/1
  Gateway Out10/1 -> F8/1
  Register23/1 -> BitBasher10/1
  Fi 2/1 -> toDsp_config102/1
  toDsp_config102/1 -> Register18/1
  Gateway Out9/1 -> F7/1
  BitBasher2/1 -> Gateway Out2/1, [F1]
  BitBasher7/1 -> Gateway Out8/1, [F6]
  toDsp_config101/1 -> Register16/1
  Fi 1/1 -> toDsp_config101/1
  Register26/1 -> BitBasher9/1
  Gateway Out13/1 -> F11/1
  Gateway Out7/1 -> F5/1
  BitBasher6/1 -> Gateway Out7/1, [F5]
  BitBasher8/1 -> Gateway Out9/1, [F7]
  BitBasher1/1 -> Gateway Out/1, [F0]
  Fi 5/1 -> toDsp_config105/1
  BitBasher9/1 -> Gateway Out10/1, [F8]
  Register21/1 -> BitBasher7/1
  BitBasher10/1 -> Gateway Out11/1, [F9]
  Fi 8/1 -> toDsp_config108/1
  toDsp_config108/1 -> Register26/1
  Fi 6/1 -> toDsp_config106/1
  toDsp_config106/1 -> Register21/1
  Fi 11/1 -> toDsp_config111/1
  toDsp_config111/1 -> Register24/1
  Fi 9/1 -> toDsp_config109/1
  toDsp_config109/1 -> Register23/1
  Register5/1 -> BitBasher1/1
  Register22/1 -> BitBasher5/1
  toDsp_config104/1 -> Register22/1
  Fi 4/1 -> toDsp_config104/1
  Register16/1 -> BitBasher2/1
  Gateway Out2/1 -> F1/1
  Register18/1 -> BitBasher3/1
  Fi 3/1 -> toDsp_config103/1
  toDsp_config103/1 -> Register17/1
  Gateway Out6/1 -> F15/1
  Fi 14/1 -> toDsp_config3/1
  toDsp_config3/1 -> Register3/1
  BitBasher15/1 -> Gateway Out15/1, [F15]
  Register2/1 -> BitBasher15/1
  Gateway Out14/1 -> F12/1
  Register3/1 -> BitBasher13/1
  BitBasher13/1 -> Gateway Out14/1, [F14]
  Gateway Out1/1 -> F14/1
  Register1/1 -> BitBasher12/1
  Register4/1 -> BitBasher16/1
  Gateway Out15/1 -> F13/1
  BitBasher16/1 -> Gateway Out1/1, [F12]
  BitBasher12/1 -> Gateway Out6/1, [F13]
  Fi 12/1 -> toDsp_config1/1
  toDsp_config1/1 -> Register4/1
  Fi 15/1 -> toDsp_config4/1
  toDsp_config4/1 -> Register2/1
  Fi 13/1 -> toDsp_config2/1
  toDsp_config2/1 -> Register1/1
